simulink library "eci_2_TLE_lib"  (R2016b)
settings: Solver=VariableStepAuto  StartTime=0.0  StopTime=10.0  RelTol=1e-3
undefined symbols (not defined in the file or in its folder): fsw_params
libraries: time_conversions_lib x1
settings Model: Creator=taylorreynolds  LastModifiedBy=Taylor

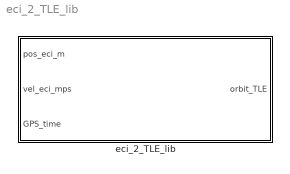
== system eci_2_TLE_lib ==
  eci_2_TLE_lib : Subsystem

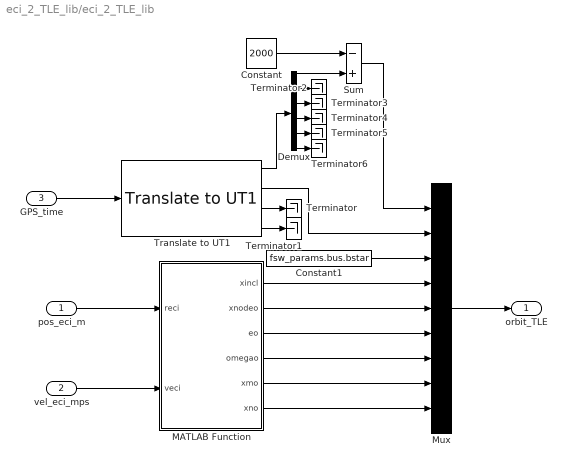
== system eci_2_TLE_lib/eci_2_TLE_lib ==
  pos_eci_m : Inport
  vel_eci_mps : Inport  Port=2
  GPS_time : Inport  Port=3
  Constant : Constant  Value=2000
  Constant1 : Constant  Value=fsw_params.bus.bstar
  Demux : Demux  Outputs=6
  MATLAB Function : MATLAB Function  TreatAsAtomicUnit=on
  Mux : Mux  Inputs=9
  Sum : Sum  Inputs=-+
  Terminator{,1..6} (7 alike) : Terminator
  Translate to UT1 : time_conversions_lib/Translate to UT1
  orbit_TLE : Outport
  wires:
  vel_eci_mps/1 -> MATLAB Function/2(veci)
  pos_eci_m/1 -> MATLAB Function/1(reci)
  MATLAB Function/6(xno) -> Mux/9
  MATLAB Function/5(xmo) -> Mux/8
  MATLAB Function/4(omegao) -> Mux/7
  MATLAB Function/3(eo) -> Mux/6
  MATLAB Function/2(xnodeo) -> Mux/5
  MATLAB Function/1(xincl) -> Mux/4
  Constant1/1 -> Mux/3
  Demux/6 -> Terminator6/1
  Demux/5 -> Terminator5/1
  Demux/4 -> Terminator4/1
  Demux/3 -> Terminator3/1
  Demux/2 -> Terminator2/1
  Demux/1 -> Sum/2
  Sum/1 -> Mux/1
  Constant/1 -> Sum/1
  Translate to UT1/1 -> Demux/1
  Translate to UT1/4 -> Terminator1/1
  Translate to UT1/3 -> Terminator/1
  Translate to UT1/2 -> Mux/2
  Mux/1 -> orbit_TLE/1
  GPS_time/1 -> Translate to UT1/1

== matlab function eci_2_TLE_lib/MATLAB Function ==
  data: xincl output size=1; xnodeo output size=1; reci input size=3; eo output size=1; omegao output size=1; xmo output size=1; veci input size=3; xno output size=1
function [xincl, xnodeo, eo, omegao, xmo, xno] = rv2tle(reci, veci)

% convert osculating position and velocity vectors
% to components of two line element set (TLE)
%   UW HuskySat-1, ADCS Subsystem
%   Updated: T. Reynolds 8.18.17

% Input

%  reci = eci position vector (meters)
%  veci = eci velocity vector (meters/second)

% Output

%  eo     = orbital eccentricity (non-dimensional)
%  xno    = mean motion (orbits per day)
%  xmo    = mean anomaly (degrees)
%  xincl  = orbital inclination (degrees)
%  omegao = argument of perigee (degrees)
%  xnodeo = right ascension of ascending node (degrees)

% Reference: Scott Campbell's Satellite Orbit Determination
%            web site www.satelliteorbitdetermination.com

% ----- Constants ----- %

pi2 = 2.0 * pi;

RAD2DEG     = 180/pi;

xke = 0.0743669161331734132;

xj3 = -2.53881d-6;

req = 6378.135;

ck2 = 5.413079d-4;

a3ovk2 = -xj3 / ck2;

xM2KM = 1e-3;
% ---------------------- %

% convert position vector to earth radii
% and velocity vector to earth radii per minute

% initialize everything
rr2     = zeros(size(reci));
vv2     = zeros(size(veci));
vk      = zeros(size(veci));
vy      = zeros(size(veci));
vz      = zeros(size(veci));
vec     = zeros(size(veci));
xincl   = 0;
xnodeo  = 0;
eo      = 0;
omegao  = 0;
xmo     = 0;
xno     = 0;

% convert to KM and KMPS
reci = reci*xM2KM;
veci = veci*xM2KM;

for i = 1:3
    rr2(i) = reci(i) / req;

    vv2(i) = 60.0d0 * veci(i) / req;

    vk(i) = vv2(i) / xke;
end

hv = cross(rr2, vk);

pl = dot(hv, hv);

vz(1) = 0.0d0;
vz(2) = 0.0d0;
vz(3) = 1.0d0;

vxh = cross(vz, hv);

if (vxh(1) == 0.0d0 && vxh(2) == 0.0d0)
    vxh(1) = 1.0d0;
end

vxhhat = vxh / norm(vxh);

rk = norm(rr2);

rdotv = dot(rr2, vv2);

rdotk = rdotv / rk;

hmag = norm(hv);

rfdotk = hmag * xke / rk;

vwrk = dot(rr2, vxhhat);

temp = vwrk / rk;

uk = acos(temp);

if (rr2(2) < 0.0d0)
    uk = pi2 - uk;
end

vz = cross(vk, hv);

for i = 1:3
    vy(i) = -1.0d0 * rr2(i) / rk;
end

for i = 1:3
    vec(i) = vz(i) + vy(i);
end

ek = norm(vec);

if (ek >= 1.0d0)
    return
end

xnodek = atan3(vxhhat(2), vxhhat(1));

temp = sqrt(hv(1) * hv(1) + hv(2) * hv(2));

xinck = atan2(temp, hv(3));

vwrk = dot(vec, vxhhat);

temp = vwrk / ek;

wk = acos(temp);

if (vec(3) < 0.0d0)
    wk = mod(pi2 - wk, pi2);
end

aodp = pl / (1.0d0 - ek * ek); %% right here - ek causes aodp to be negative, inducing complex numbers
% throughout the rest of the code. Should have ek < 1. Fix here.
aodp = real(aodp);

xn = xke * aodp^(-1.5);


% in the first loop the osculating elements rk, uk, xnodek, xinck, rdotk,
% and rfdotk are used as anchors to find the corresponding final sgp4
% mean elements r, u, xnodeo, xincl, rdot, and rfdot. several other final
% mean values based on these are also found: betal, cosio, sinio, theta2,
% cos2u, sin2u, x3thm1, x7thm1, x1mth2. in addition, the osculating values
% initially held by aodp, pl, and xn are replaced by intermediate
% (not osculating and not mean) values used by sgp4. the loop converges
% on the value of pl in about four iterations.

% seed value for first loop

xincl = xinck;

u = uk;

for i = 1:1:20

    a2 = pl;

    betal = sqrt(pl / aodp);

    temp1 = ck2 / pl;

    temp2 = temp1 / pl;

    cosio = cos(xincl);

    sinio = sin(xincl);

    sin2u = sin(2.0d0 * u);

    cos2u = cos(2.0d0 * u);

    theta2 = cosio * cosio;

    x3thm1 = 3.0d0 * theta2 - 1.0d0;

    x1mth2 = 1.0d0 - theta2;

    x7thm1 = 7.0d0 * theta2 - 1.0d0;

    r = (rk - 0.5d0 * temp1 * x1mth2 * cos2u) ...
        / (1.0d0 - 1.5d0 * temp2 * betal * x3thm1);

    u = uk + 0.25d0 * temp2 * x7thm1 * sin2u;

    xnodeo = xnodek - 1.5d0 * temp2 * cosio * sin2u;

    xincl = xinck - 1.5d0 * temp2 * cosio * sinio * cos2u;

    rdot = rdotk + xn * temp1 * x1mth2 * sin2u;

    rfdot = rfdotk - xn * temp1 * (x1mth2 * cos2u + 1.5d0 * x3thm1);

    temp = r * rfdot / xke;

    pl = temp * temp;

    temp = 2.0d0 / r - (rdot * rdot + rfdot * rfdot) / (xke * xke);

    aodp = 1.0d0 / temp;

    xn = xke * aodp ^ (-1.5d0);

    if (abs(a2 - pl) < 1.0d-13)
        break
    end

%     if (i == 20)
%         fprintf('\n20 iterations in first loop');
%     end
end

% the next values are calculated from constants and a combination of mean
% and intermediate quantities from the first loop. these values all remain
% fixed and are used in the second loop.

% preliminary values for the second loop

ecose = 1.0d0 - r / aodp;

esine = r * rdot / (xke * sqrt(aodp));

elsq = 1.0d0 - pl / aodp;

xlcof = 0.125d0 * a3ovk2 * sinio * (3.0d0 + 5.0d0 * cosio) / (1.0d0 + cosio);

aycof = 0.25d0 * a3ovk2 * sinio;

temp1 = esine / (1.0d0 + sqrt(1.0d0 - elsq));

cosu = cos(u);

sinu = sin(u);

% the second loop normally converges in about six iterations to the final
% mean value for the eccentricity, eo. the mean perigee, omegao, is also
% determined. cosepw and sinepw are found to twelve decimal places and
% are used to calculate an intermediate value for the eccentric anomaly,
% temp2. temp2 is then used in kepler's equation to find an intermediate
% value for the true longitude, capu.

% seed values for loop

eo = sqrt(elsq);

omegao = wk;

axn = eo * cos(omegao);

for i = 1:1:20

    a2 = eo;

    beta = 1.0d0 - eo * eo;

    temp = 1.0d0 / (aodp * beta);

    aynl = temp * aycof;

    ayn = eo * sin(omegao) + aynl;

    cosepw = r * cosu / aodp + axn - ayn * temp1;

    sinepw = r * sinu / aodp + ayn + axn * temp1;

    axn = cosepw * ecose + sinepw * esine;

    ayn = sinepw * ecose - cosepw * esine;

    omegao = mod(atan2(ayn - aynl, axn), pi2);

    if (eo > 0.5d0)
        eo = 0.9d0 * eo + 0.1d0 * (axn / cos(omegao));
    else
        eo = axn / cos(omegao);
    end

    if (eo > 0.999d0)
        eo = 0.999d0;
    end

    if (abs(a2 - eo) < 1.0d-9)
        break
    end

%     if (i == 20)
%         fprintf('\n20 iterations in second loop');
%     end
end

temp2 = atan2(sinepw, cosepw);

capu = temp2 - esine;

xll = temp * xlcof * axn;

% xll adjusts the intermediate true longitude
% capu, to the mean true longitude, xl

xl = capu - xll;

xmo = mod(xl - omegao, pi2);

% the third loop usually converges after three iterations to the
% mean semi-major axis, a1, which is then used to find the mean motion, xno

a0 = aodp;

a1 = a0;

beta2 = sqrt(beta);

temp = 1.5d0 * ck2 * x3thm1 / (beta * beta2);

for i = 1:1:20

    a2 = a1;

    d0 = temp / (a0 * a0);

    a0 = aodp * (1.0d0 - d0);

    d1 = temp / (a1 * a1);

    a1 = a0 / (1.0d0 - d1 / 3.0d0 - d1 * d1 - 134.0d0 * d1 * d1 * d1 / 81.0d0);

    if (abs(a2 - a1) < 1.0d-13)
        break
    end

%     if (i == 20)
%         fprintf('\n20 iterations in third loop');
%     end
end

xno = xke * a1 ^ (-1.5d0);

xno = xno / (pi2 / 1440.0d0);

% Convert to right units
xmo     = RAD2DEG*xmo;
xincl   = RAD2DEG*xincl;
omegao  = RAD2DEG*omegao;
xnodeo  = RAD2DEG*xnodeo;

end % function
